simulink model "U"  (R2013a)
settings: Solver=ode45  StartTime=0.0  StopTime=1.0  RelTol=1e-3
libraries: powerlib x9, electricdrivelib x1, fl_lib x1, simulink x1
settings Model: Creator=hp  LastModifiedBy=hp

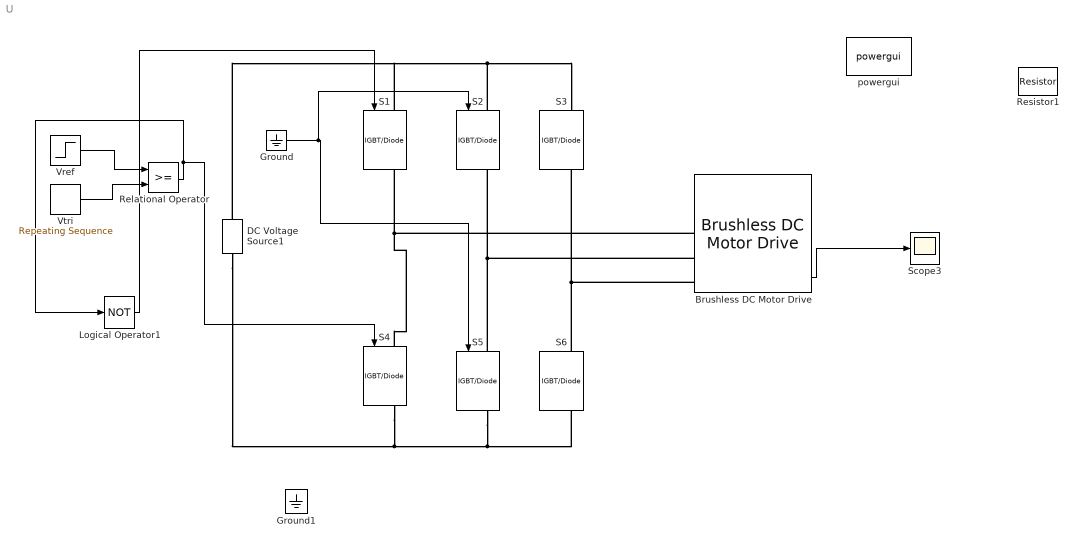
== system U ==
  Brushless DC Motor Drive : electricdrivelib/AC drives/Brushless DC Motor Drive  showMaskWarnings=on  AverageValue=off  MechanicalLoad=Torque Tm  driveType=AC7
  DC Voltage Source1 : powerlib/Electrical Sources/DC Voltage Source  Amplitude=240  Measurements=None
  Ground : Ground
  Ground1 : powerlib/Elements/Ground  LConnTagsString=a
  Logical Operator1 : Logic  Operator=NOT  AllPortsSameDT=off  OutDataTypeStr=boolean
  Relational Operator : RelationalOperator  OutDataTypeStr=boolean
  Resistor1 : fl_lib/Electrical/Electrical Elements/Resistor  R=1 Ohm  i_Log=off  v_Log=off  LocalVarNames=|i|v  LocalVarDescs=|i|v  LocalVarLogging=[0 0]
  S{1..6} (6 alike) : powerlib/Power Electronics/IGBT//Diode  Ron=1e-3  Rs=1e5  Cs=inf  Measurements=on
  Scope3 : Scope
      settings: SaveName=IC
  "Vref " : Step  Time=0  After=150  SampleTime=0
  Vtri : simulink/Sources/Repeating Sequence  rep_seq_t=[0 (1/2) 1]*0.001  rep_seq_y="[-1  1 -1] *240"
  powergui : powerlib/powergui  Priority=1  SimulationMode=Discrete  SolverType=Tustin  SampleTime=1e-6  frequency=60  SPID=off  DisableSnubberDevices=off  DisableRonSwitches=off  DisableVfSwitches=off  SwTol=0  Interpol=off  DisplayEquations=off  frequencyindice=0  Pbase=100e6  ErrMax=1e-4  Iterations=50  UnitsV=kV  UnitsW=MW  FunctionMessages=off  echomessages=off  HookPort=off  EnableUseOfTLC=off  x0status=blocks  RestoreLinks=warning  ResistiveCurrentMeasurement=off  Frange=[0:2:500]  Ylog=off  Xlog=on  ShowGrid=off  save=off  variable=ZData  ZoomFFT=off  StartTime=0.0  cycles=1  DisplayStyle=1  fundamental=60  FreqAxis=off  MaxFrequency=1000  frequencyindicesteady=1  RmsSteady=1  display=off  Ts=0  methode=off
  wires:
  Vtri/1 -> Relational Operator/2
  "Vref "/1 -> Relational Operator/1
  Relational Operator/1 -> S4/1, Logical Operator1/1
  Ground/1 -> S2/1, S5/1
  Logical Operator1/1 -> S1/1
  Brushless DC Motor Drive/4 -> Scope3/1
  connections:
  S6/LConn1 -- Brushless DC Motor Drive/LConn3 -- S3/RConn1
  DC Voltage Source1/LConn1 -- S4/RConn1 -- S5/RConn1 -- S6/RConn1
  S2/LConn1 -- S3/LConn1 -- DC Voltage Source1/RConn1 -- S1/LConn1
  S4/LConn1 -- Brushless DC Motor Drive/LConn1 -- S1/RConn1
  S5/LConn1 -- Brushless DC Motor Drive/LConn2 -- S2/RConn1
